simulink model "TV_2018_HIL"  (R2016a)
settings: Solver=FixedStepAuto  StartTime=0.0  StopTime=inf  FixedStep=0.001  RelTol=1e-3
PreLoadFcn:
  | TV_2017_parameters
values from neighbouring files (symbols this model uses):
  battery_voltage = single(530)    [HIL_parameters.m]    (also in HIL_parameters_2018.m; TV_2017_parameters.m; TV_2017_parameters_VD.m)
  car_params = Simulink_Car_params    [HIL_parameters.m]    (also in HIL_parameters_2018.m; TV_2017_parameters.m; TV_2017_parameters_VD.m)
  i_Diff = 16    [HIL_parameters.m]    (also in HIL_parameters_2018.m; TV_2017_parameters.m)
  Kp = 1    [HIL_parameters.m]    (also in HIL_parameters_2018.m; TV_2017_parameters.m; TV_2017_parameters_VD.m)
  motor_data = struct    [HIL_parameters.m]    (also in HIL_parameters_2018.m; TV_2017_parameters.m)
  powerLimitControl = Simulink_el    [HIL_parameters.m]    (also in HIL_parameters_2018.m; TV_2017_parameters.m; TV_2017_parameters_VD.m)
  settings = Simulink_Settings    [HIL_parameters.m]    (also in HIL_parameters_2018.m; TV_2017_parameters.m; TV_2017_parameters_VD.m)
  SpdC_BCC = 0    [HIL_parameters.m]    (also in HIL_parameters_2018.m; TV_2017_parameters.m; TV_2017_parameters_VD.m)
  Speed_Neg_sat = -21    [HIL_parameters.m]    (also in HIL_parameters_2018.m; TV_2017_parameters.m; TV_2017_parameters_VD.m)
  Speed_Pos_sat = 21    [HIL_parameters.m]    (also in HIL_parameters_2018.m; TV_2017_parameters.m; TV_2017_parameters_VD.m)
  SteeringAngleFL = [-23.80 -22.65 -21.50 -20.34 -19.18 -18.03 -16.86 -15.70 -14.53 -13.35 -12.18 -10.99 -9.80 -8.61 -7.40 -6.19 -4.97 -3.75 -2.51 -1.26 0 1.27 2.56 3.85 5.17 6.50 7.84 9.21 10.59 12.00 13.42 14.88 16.36 17.87 19.41 20.99 22.61 24.26 25.97 27.73 29.54]    [CarSetupAnalysis2018.m]    (also in HIL_parameters_2018.m; TV_2017_parameters.m; TV_2017_parameters_VD.m = [-24.129 -22.950 -21.772 -20.593 -19.413 -18.232 -17.050 -15)
  SteeringAngleFR = [-29.54 -27.73 -25.97 -24.26 -22.61 -20.99 -19.41 -17.87 -16.36 -14.88 -13.42 -12.00 -10.59 -9.21 -7.84 -6.50 -5.17 -3.85 -2.56 -1.27 0 1.26 2.51 3.75 4.97 6.19 7.40 8.61 9.80 10.99 12.18 13.35 14.53 15.70 16.86 18.03 19.18 20.34 21.50 22.65 23.80]    [CarSetupAnalysis2018.m]    (also in HIL_parameters_2018.m; TV_2017_parameters.m; TV_2017_parameters_VD.m = [-29.3050 -27.5340 -25.8140 -24.1410 -22.5110 -20.9180 -19.3)
  SteeringWhAngle = [-105 -99.75 -94.5 -89.25 -84 -78.75 -73.5 -68.25 -63 -57.75 -52.5 -47.25 -42 -36.75 -31.5 -26.25 -21.0 -15.75 -10.5 -5.25 0.0 5.25 10.50 15.75 21.00 26.25 31.50 36.75 42.00 47.25 52.50 57.75  63.00 68.25 73.50 78.75 84.00 89.25 94.50 99.75 105.00]    [TV_2017_parameters_VD.m]
  Tn_n = 0    [HIL_parameters.m]    (also in HIL_parameters_2018.m; TV_2017_parameters.m; TV_2017_parameters_VD.m)
  tractionControl = Simulink_tc    [HIL_parameters.m]    (also in HIL_parameters_2018.m; IterativeTractionControlTuning.m; TV_2017_parameters.m; TV_2017_parameters_VD.m)
  yawMomentGenerator = struct    [HIL_parameters.m]    (also in HIL_parameters_2018.m = Simulink_yawRate2; TV_2017_parameters.m = Simulink_yawRate2)
  yawRateControl = Simulink_yawRate    [HIL_parameters.m]    (also in HIL_parameters_2018.m; TV_2017_parameters.m; TV_2017_parameters_VD.m)
undefined symbols (not defined in the file or in its folder): canChannel, DiscIntNeverNeededParam, magnitude, speedEstimation, TC_Decr_Gas, TC_Derivative, TC_Incr_Gas, TC_On, TC_Relay_Off, TC_Relay_On
libraries: CarMaker4SL x366, simulink_extras x63, canmsglib x55, canlib x41, simulink x37, dspfdesign x2, sldrtlib x1
(part 7 of 15)

== system TV_2018_HIL/CarMaker/IPG Vehicle3/CarAndTrailer/Forces/Tires ==
  note: The TireXX_Out signals will only be used if FileIdent is "CarMaker-Tire-CM4SL" in the tire parameter file!
      | An example parameter file can be found in Data/Tire/DT_CM4SL_UserTire.
  Sync_In : Inport
  TireFL_In : Inport  Port=2
  TireFR_In : Inport  Port=3
  TireRL_In : Inport  Port=4
  TireRR_In : Inport  Port=5
  Bus Creator{1..4} (4 alike) : BusCreator  Inputs=11
  Demux{1..3,8} (4 alike) : Demux  Outputs=7
  Scope : Scope
  TireFL : Subsystem
  TireFR : Subsystem
  TireRL : Subsystem
  TireRR : Subsystem
  TireFL_Out : Outport
  TireFR_Out : Outport  Port=2
  TireRL_Out : Outport  Port=3
  TireRR_Out : Outport  Port=4
  wires:
  Sync_In/1 -> TireRR/1(Sync_In), TireRL/1(Sync_In), TireFR/1(Sync_In), TireFL/1(Sync_In)
  Bus Creator4/1 -> TireRR_Out/1
  Bus Creator2/1 -> TireRL_Out/1
  Bus Creator1/1 -> TireFR_Out/1
  Demux3/5 -> TireRR/6(Rim_turnv)  "Tire_In Rim_turnv"
  Demux3/4 -> TireRR/5(Rim_rotv)  "Tire_In Rim_rotv"
  Demux3/1 -> TireRR/2(Load)  "Tire_In Load"
  Demux3/7 -> TireRR/8(muRoad)  "Tire_In mu"
  Demux3/6 -> TireRR/7(InclinAngle)  "Tire_In Camber"
  Demux3/2 -> TireRR/3(vxtrans)  "Tire_In vxtrans"
  Demux3/3 -> TireRR/4(vytrans)  "Tire_In vytrans"
  TireRR/11(AlignTrq) -> Bus Creator4/11  "Tire_Out AlignTrq"
  TireRR/10(RollResist) -> Bus Creator4/10  "Tire_Out RollResist"
  TireRR/9(OverturnTrq) -> Bus Creator4/9  "Tire_Out OverturnTrq"
  TireRR/8(LoadFrc) -> Bus Creator4/8  "Tire_Out LoadFrc"
  TireRR/7(SideFrc) -> Bus Creator4/7  "Tire_Out SideFrc"
  TireRR/6(LongFrc) -> Bus Creator4/6  "Tire_Out LongFrc"
  TireRR/5(vBelt) -> Bus Creator4/5  "Tire_Out vBelt"
  TireRR/4(rBelt_eff) -> Bus Creator4/4  "Tire_Out rBelt_eff"
  TireRR/3(TurnSlp) -> Bus Creator4/3  "Tire_Out TurnSlp"
  TireRR/1(Slp) -> Bus Creator4/1  "Tire_Out Slp"
  TireRR/2(Alpha) -> Bus Creator4/2  "Tire_Out Alpha"
  Demux2/5 -> TireRL/6(Rim_turnv)  "Tire_In Rim_turnv"
  Demux2/4 -> TireRL/5(Rim_rotv)  "Tire_In Rim_rotv"
  Demux2/1 -> TireRL/2(Load)  "Tire_In Load"
  Demux2/7 -> TireRL/8(muRoad)  "Tire_In mu"
  Demux2/6 -> TireRL/7(InclinAngle)  "Tire_In Camber"
  Demux2/2 -> TireRL/3(vxtrans)  "Tire_In vxtrans"
  Demux2/3 -> TireRL/4(vytrans)  "Tire_In vytrans"
  TireRL/11(AlignTrq) -> Bus Creator2/11  "Tire_Out AlignTrq"
  TireRL/10(RollResist) -> Bus Creator2/10  "Tire_Out RollResist"
  TireRL/9(OverturnTrq) -> Bus Creator2/9  "Tire_Out OverturnTrq"
  TireRL/8(LoadFrc) -> Bus Creator2/8  "Tire_Out LoadFrc"
  TireRL/7(SideFrc) -> Bus Creator2/7  "Tire_Out SideFrc"
  TireRL/6(LongFrc) -> Bus Creator2/6  "Tire_Out LongFrc"
  TireRL/5(vBelt) -> Bus Creator2/5  "Tire_Out vBelt"
  TireRL/4(rBelt_eff) -> Bus Creator2/4  "Tire_Out rBelt_eff"
  TireRL/3(TurnSlp) -> Bus Creator2/3  "Tire_Out TurnSlp"
  TireRL/1(Slp) -> Bus Creator2/1  "Tire_Out Slp"
  TireRL/2(Alpha) -> Bus Creator2/2  "Tire_Out Alpha"
  Demux1/5 -> TireFR/6(Rim_turnv)  "Tire_In Rim_turnv"
  Demux1/4 -> TireFR/5(Rim_rotv)  "Tire_In Rim_rotv"
  Demux1/1 -> TireFR/2(Load)  "Tire_In Load"
  Demux1/7 -> TireFR/8(muRoad)  "Tire_In mu"
  Demux1/6 -> TireFR/7(InclinAngle)  "Tire_In Camber"
  Demux1/2 -> TireFR/3(vxtrans)  "Tire_In vxtrans"
  Demux1/3 -> TireFR/4(vytrans)  "Tire_In vytrans"
  TireFR/11(AlignTrq) -> Bus Creator1/11  "Tire_Out AlignTrq"
  TireFR/10(RollResist) -> Bus Creator1/10  "Tire_Out RollResist"
  TireFR/9(OverturnTrq) -> Bus Creator1/9  "Tire_Out OverturnTrq"
  TireFR/8(LoadFrc) -> Bus Creator1/8  "Tire_Out LoadFrc"
  TireFR/7(SideFrc) -> Bus Creator1/7  "Tire_Out SideFrc"
  TireFR/6(LongFrc) -> Bus Creator1/6  "Tire_Out LongFrc"
  TireFR/5(vBelt) -> Bus Creator1/5  "Tire_Out vBelt"
  TireFR/4(rBelt_eff) -> Bus Creator1/4  "Tire_Out rBelt_eff"
  TireFR/3(TurnSlp) -> Bus Creator1/3  "Tire_Out TurnSlp"
  TireFR/1(Slp) -> Bus Creator1/1  "Tire_Out Slp"
  TireFR/2(Alpha) -> Bus Creator1/2  "Tire_Out Alpha"
  Demux8/5 -> TireFL/6(Rim_turnv)  "Tire_In Rim_turnv"
  Demux8/4 -> TireFL/5(Rim_rotv)  "Tire_In Rim_rotv"
  TireFL_In/1 -> Demux8/1
  Demux8/1 -> TireFL/2(Load)  "Tire_In Load"
  Demux8/7 -> Scope/1, TireFL/8(muRoad)  "Tire_In mu"
  Demux8/6 -> TireFL/7(InclinAngle)  "Tire_In Camber"
  Demux8/2 -> TireFL/3(vxtrans)  "Tire_In vxtrans"
  Demux8/3 -> TireFL/4(vytrans)  "Tire_In vytrans"
  TireFL/11(AlignTrq) -> Bus Creator3/11  "Tire_Out AlignTrq"
  TireFL/10(RollResist) -> Bus Creator3/10  "Tire_Out RollResist"
  TireFL/9(OverturnTrq) -> Bus Creator3/9  "Tire_Out OverturnTrq"
  TireFL/8(LoadFrc) -> Bus Creator3/8  "Tire_Out LoadFrc"
  TireFL/7(SideFrc) -> Bus Creator3/7  "Tire_Out SideFrc"
  TireFL/6(LongFrc) -> Bus Creator3/6  "Tire_Out LongFrc"
  TireFL/5(vBelt) -> Bus Creator3/5  "Tire_Out vBelt"
  TireFL/4(rBelt_eff) -> Bus Creator3/4  "Tire_Out rBelt_eff"
  TireFL/3(TurnSlp) -> Bus Creator3/3  "Tire_Out TurnSlp"
  TireFL/1(Slp) -> Bus Creator3/1  "Tire_Out Slp"
  TireFL/2(Alpha) -> Bus Creator3/2  "Tire_Out Alpha"
  Bus Creator3/1 -> TireFL_Out/1
  TireFR_In/1 -> Demux1/1
  TireRL_In/1 -> Demux2/1
  TireRR_In/1 -> Demux3/1

== system TV_2018_HIL/CarMaker/IPG Vehicle3/CarAndTrailer/Forces/Vehicle Forces ==
  Sync_In : Inport
  Aero R18 prelim : Subsystem
  Bus Creator1 : BusCreator  Inputs=12
  Bus Creator8 : BusCreator  Inputs=16
  BusCreator1 : BusCreator  Inputs=4
  BusCreator2 : BusCreator  Inputs=9
  Demux : Demux  Outputs=16
  Demux1 : Demux  Outputs=12
  Demux2 : Demux  Outputs=13
  Forces : S-Function  FunctionName=CM_Sfun  Parameters='Forces'  SFunctionDeploymentMode=off  EnableBusSupport=off
  Terminator : Terminator
  Sync_Out : Outport
  Car.Virtual : Outport  Port=2
  Car.Aero : Outport  Port=3
  Car.Load : Outport  Port=4
  wires:
  BusCreator1/1 -> Terminator/1  "Aero IF (in)"
  Demux/16 -> Bus Creator8/16  "Car Load_3 tz"
  Demux/15 -> Bus Creator8/15  "Car Load_3 ty"
  Demux/14 -> Bus Creator8/14  "Car Load_3 tx"
  Demux/13 -> Bus Creator8/13  "Car Load_3 mass"
  Demux1/12 -> Bus Creator1/12  "Car Virtual Trq_0 z"
  Demux1/11 -> Bus Creator1/11  "Car Virtual Trq_0 y"
  Demux1/10 -> Bus Creator1/10  "Car Virtual Trq_0 x"
  Demux1/9 -> Bus Creator1/9  "Car Virtual Trq_1 z"
  Demux1/8 -> Bus Creator1/8  "Car Virtual Trq_1 y"
  Demux1/7 -> Bus Creator1/7  "Car Virtual Trq_1 x"
  Demux1/6 -> Bus Creator1/6  "Car Virtual Frc_0 z"
  Demux1/5 -> Bus Creator1/5  "Car Virtual Frc_0 y"
  Demux1/4 -> Bus Creator1/4  "Car Virtual Frc_0 x"
  Sync_In/1 -> Forces/1
  Forces/1 -> Sync_Out/1
  BusCreator2/1 -> Car.Aero/1
  Demux1/1 -> Bus Creator1/1  "Car Virtual Frc_1 x"
  Demux1/2 -> Bus Creator1/2  "Car Virtual Frc_1 y"
  Demux1/3 -> Bus Creator1/3  "Car Virtual Frc_1 z"
  Forces/3 -> Demux2/1
  Forces/2 -> Demux1/1
  Bus Creator1/1 -> Car.Virtual/1
  Bus Creator8/1 -> Car.Load/1
  Demux/1 -> Bus Creator8/1  "Car Load_0 mass"
  Demux/2 -> Bus Creator8/2  "Car Load_0 tx"
  Demux/3 -> Bus Creator8/3  "Car Load_0 ty"
  Demux/4 -> Bus Creator8/4  "Car Load_0 tz"
  Demux/5 -> Bus Creator8/5  "Car Load_1 mass"
  Demux/6 -> Bus Creator8/6  "Car Load_1 tx"
  Demux/7 -> Bus Creator8/7  "Car Load_1 ty"
  Demux/8 -> Bus Creator8/8  "Car Load_1 tz"
  Demux/9 -> Bus Creator8/9  "Car Load_2 mass"
  Demux/10 -> Bus Creator8/10  "Car Load_2 tx"
  Demux/11 -> Bus Creator8/11  "Car Load_2 ty"
  Demux/12 -> Bus Creator8/12  "Car Load_2 tz"
  Forces/4 -> Demux/1
  Demux2/1 -> Aero R18 prelim/1(car Aero ApproachVel_1 x)  "car Aero ApproachVel_1 x"
  Demux2/2 -> Aero R18 prelim/2(car Aero ApproachVel_1 y)  "car Aero ApproachVel_1 y"
  Demux2/3 -> Aero R18 prelim/3(car Aero ApproachVel_1 z)  "car Aero ApproachVel_1 z"
  Demux2/4 -> Aero R18 prelim/4(car Aero tau_1)  "car Aero tau_1"
  Demux2/5 -> Aero R18 prelim/5(car Aero PoA_1 x)  "car Aero PoA_1 x"
  Demux2/6 -> Aero R18 prelim/6(car Aero PoA_1 y)  "car Aero PoA_1 y"
  Demux2/7 -> Aero R18 prelim/7(car Aero PoA_1 z)  "car Aero PoA_1 z"
  Demux2/8 -> Aero R18 prelim/8(car Aero Frc_1 x)  "car Aero Frc_1 x"
  Demux2/9 -> Aero R18 prelim/9(car Aero Frc_1 y)  "car Aero Frc_1 y"
  Demux2/10 -> Aero R18 prelim/10(car Aero Frc_1 z)  "car Aero Frc_1 z"
  Demux2/11 -> Aero R18 prelim/11(car Aero Trq_1 x)  "car Aero Trq_1 x"
  Demux2/12 -> Aero R18 prelim/12(car Aero Trq_1 y)  "car Aero Trq_1 y"
  Demux2/13 -> Aero R18 prelim/13(car Aero Trq_1 z)  "car Aero Trq_1 z"
  Aero R18 prelim/7(car Aero PoA_1 z_R18) -> BusCreator2/3
  Aero R18 prelim/8(car Aero Frc_1 x_R18) -> BusCreator2/4
  Aero R18 prelim/9(car Aero Frc_1 y_R18) -> BusCreator2/5
  Aero R18 prelim/10(car Aero Frc_1 z_R18) -> BusCreator2/6
  Aero R18 prelim/11(car Aero Trq_1 x_R18) -> BusCreator2/7
  Aero R18 prelim/12(car Aero Trq_1 y_R18) -> BusCreator2/8
  Aero R18 prelim/13(car Aero Trq_1 z_R18) -> BusCreator2/9
  Aero R18 prelim/5(car Aero PoA_1 x_R18) -> BusCreator2/1
  Aero R18 prelim/6(car Aero PoA_1 y_R18) -> BusCreator2/2
  Aero R18 prelim/4(car Aero tau_1_R18) -> BusCreator1/4
  Aero R18 prelim/3(car Aero ApproachVel_1 z_R18) -> BusCreator1/3
  Aero R18 prelim/2(car Aero ApproachVel_1 y_R18) -> BusCreator1/2
  Aero R18 prelim/1(car Aero ApproachVel_1 x_R18) -> BusCreator1/1

== system TV_2018_HIL/CarMaker/IPG Vehicle3/CarAndTrailer/Trailer/CreateBus Car.Hitch.FrcTrq ==
  In1 : Inport
  Bus Creator7 : BusCreator  Inputs=6
  Demux7 : Demux  Outputs=6
  Out1 : Outport
  wires:
  In1/1 -> Demux7/1
  Bus Creator7/1 -> Out1/1
  Demux7/6 -> Bus Creator7/6  "Car Hitch Trq2Car z"
  Demux7/5 -> Bus Creator7/5  "Car Hitch Trq2Car y"
  Demux7/4 -> Bus Creator7/4  "Car Hitch Trq2Car x"
  Demux7/3 -> Bus Creator7/3  "Car Hitch Frc2Car z"
  Demux7/2 -> Bus Creator7/2  "Car Hitch Frc2Car y"
  Demux7/1 -> Bus Creator7/1  "Car Hitch Frc2Car x"

== system TV_2018_HIL/CarMaker/IPG Vehicle3/CarAndTrailer/Trailer/CreateBus Vhcl.Motion ==
  In1 : Inport
  BusCreator : BusCreator  Inputs=15
  Demux : Demux  Outputs=15
  Out1 : Outport
  wires:
  Demux/15 -> BusCreator/15  "Vhcl YawAcc"
  Demux/14 -> BusCreator/14  "Vhcl YawVel"
  Demux/13 -> BusCreator/13  "Vhcl Yaw"
  Demux/12 -> BusCreator/12  "Vhcl PitchAcc"
  Demux/11 -> BusCreator/11  "Vhcl PitchVel"
  Demux/10 -> BusCreator/10  "Vhcl Pitch"
  Demux/9 -> BusCreator/9  "Vhcl RollAcc"
  Demux/8 -> BusCreator/8  "Vhcl RollVel"
  Demux/7 -> BusCreator/7  "Vhcl Roll"
  Demux/6 -> BusCreator/6  "Vhcl Hitch_Pos z"
  Demux/5 -> BusCreator/5  "Vhcl Hitch_Pos y"
  Demux/4 -> BusCreator/4  "Vhcl Hitch_Pos x"
  Demux/3 -> BusCreator/3  "Vhcl sRoad"
  Demux/2 -> BusCreator/2  "Vhcl Distance"
  Demux/1 -> BusCreator/1  "Vhcl v"
  In1/1 -> Demux/1
  BusCreator/1 -> Out1/1

== system TV_2018_HIL/CarMaker/IPG Vehicle3/CarAndTrailer/Trailer/CreateBus Vhcl.PoI ==
  In1 : Inport
  Bus Creator3 : BusCreator  Inputs=18
  Demux3 : Demux  Outputs=18
  Out1 : Outport
  wires:
  Demux3/18 -> Bus Creator3/18  "Vhcl PoI_GCS Elev"
  Demux3/17 -> Bus Creator3/17  "Vhcl PoI_GCS Lat"
  Demux3/16 -> Bus Creator3/16  "Vhcl PoI_GCS Long"
  Demux3/15 -> Bus Creator3/15  "Vhcl PoI_Acc_1 z"
  Demux3/14 -> Bus Creator3/14  "Vhcl PoI_Acc_1 y"
  Demux3/13 -> Bus Creator3/13  "Vhcl PoI_Acc_1 x"
  Demux3/12 -> Bus Creator3/12  "Vhcl PoI_Vel_1 z"
  Demux3/11 -> Bus Creator3/11  "Vhcl PoI_Vel_1 y"
  Demux3/10 -> Bus Creator3/10  "Vhcl PoI_Vel_1 x"
  Demux3/9 -> Bus Creator3/9  "Vhcl PoI_Acc z"
  Demux3/8 -> Bus Creator3/8  "Vhcl PoI_Acc y"
  Demux3/7 -> Bus Creator3/7  "Vhcl PoI_Acc x"
  Demux3/6 -> Bus Creator3/6  "Vhcl PoI_Vel z"
  Demux3/5 -> Bus Creator3/5  "Vhcl PoI_Vel y"
  Demux3/4 -> Bus Creator3/4  "Vhcl PoI_Vel x"
  Demux3/3 -> Bus Creator3/3  "Vhcl PoI_Pos z"
  Demux3/2 -> Bus Creator3/2  "Vhcl PoI_Pos y"
  In1/1 -> Demux3/1
  Bus Creator3/1 -> Out1/1
  Demux3/1 -> Bus Creator3/1  "Vhcl PoI_Pos x"

== system TV_2018_HIL/CarMaker/IPG Vehicle3/CarAndTrailer/Trailer/CreateBus Vhcl.Steering ==
  In1 : Inport
  Bus Creator3 : BusCreator  Inputs=4
  Demux : Demux
  Out1 : Outport
  wires:
  Bus Creator3/1 -> Out1/1
  Demux/1 -> Bus Creator3/1  "Vhcl Steering Ang"
  Demux/3 -> Bus Creator3/3  "Vhcl Steering AngAcc"
  Demux/2 -> Bus Creator3/2  "Vhcl Steering AngVel"
  Demux/4 -> Bus Creator3/4  "Vhcl Steering Trq"
  In1/1 -> Demux/1

== system TV_2018_HIL/CarMaker/IPG Vehicle3/CarAndTrailer/Trailer/CreateBus Vhcl.Wheel.FL ==
  In1 : Inport
  Bus Creator3 : BusCreator  Inputs=14
  Demux3 : Demux  Outputs=14
  Out1 : Outport
  wires:
  Demux3/14 -> Bus Creator3/14  "Vhcl Wheel FL Trq_WhlBearing"
  Demux3/13 -> Bus Creator3/13  "Vhcl Wheel FL Trq_T2W"
  Demux3/12 -> Bus Creator3/12  "Vhcl Wheel FL SideSlip"
  Demux3/11 -> Bus Creator3/11  "Vhcl Wheel FL LongSlip"
  Demux3/10 -> Bus Creator3/10  "Vhcl Wheel FL vBelt"
  Demux3/9 -> Bus Creator3/9  "Vhcl Wheel FL Fz"
  Demux3/8 -> Bus Creator3/8  "Vhcl Wheel FL Fy"
  Demux3/7 -> Bus Creator3/7  "Vhcl Wheel FL Fx"
  Demux3/6 -> Bus Creator3/6  "Vhcl Wheel FL r_zxy z"
  Demux3/5 -> Bus Creator3/5  "Vhcl Wheel FL r_zxy y"
  Demux3/4 -> Bus Creator3/4  "Vhcl Wheel FL r_zxy x"
  Demux3/3 -> Bus Creator3/3  "Vhcl Wheel FL t z"
  Demux3/2 -> Bus Creator3/2  "Vhcl Wheel FL t y"
  In1/1 -> Demux3/1
  Bus Creator3/1 -> Out1/1
  Demux3/1 -> Bus Creator3/1  "Vhcl Wheel FL t x"

== system TV_2018_HIL/CarMaker/IPG Vehicle3/CarAndTrailer/Trailer/CreateBus Vhcl.Wheel.FR ==
  In1 : Inport
  Bus Creator3 : BusCreator  Inputs=14
  Demux3 : Demux  Outputs=14
  Out1 : Outport
  wires:
  Demux3/14 -> Bus Creator3/14  "Vhcl Wheel FR Trq_WhlBearing"
  Demux3/13 -> Bus Creator3/13  "Vhcl Wheel FR Trq_T2W"
  Demux3/12 -> Bus Creator3/12  "Vhcl Wheel FR SideSlip"
  Demux3/11 -> Bus Creator3/11  "Vhcl Wheel FR LongSlip"
  Demux3/10 -> Bus Creator3/10  "Vhcl Wheel FR vBelt"
  Demux3/9 -> Bus Creator3/9  "Vhcl Wheel FR Fz"
  Demux3/8 -> Bus Creator3/8  "Vhcl Wheel FR Fy"
  Demux3/7 -> Bus Creator3/7  "Vhcl Wheel FR Fx"
  Demux3/6 -> Bus Creator3/6  "Vhcl Wheel FR r_zxy z"
  Demux3/5 -> Bus Creator3/5  "Vhcl Wheel FR r_zxy y"
  Demux3/4 -> Bus Creator3/4  "Vhcl Wheel FR r_zxy x"
  Demux3/3 -> Bus Creator3/3  "Vhcl Wheel FR t z"
  Demux3/2 -> Bus Creator3/2  "Vhcl Wheel FR t y"
  In1/1 -> Demux3/1
  Bus Creator3/1 -> Out1/1
  Demux3/1 -> Bus Creator3/1  "Vhcl Wheel FR t x"

== system TV_2018_HIL/CarMaker/IPG Vehicle3/CarAndTrailer/Trailer/CreateBus Vhcl.Wheel.RL ==
  In1 : Inport
  Bus Creator3 : BusCreator  Inputs=14
  Demux3 : Demux  Outputs=14
  Out1 : Outport
  wires:
  Demux3/14 -> Bus Creator3/14  "Vhcl Wheel RL Trq_WhlBearing"
  Demux3/13 -> Bus Creator3/13  "Vhcl Wheel RL Trq_T2W"
  Demux3/12 -> Bus Creator3/12  "Vhcl Wheel RL SideSlip"
  Demux3/11 -> Bus Creator3/11  "Vhcl Wheel RL LongSlip"
  Demux3/10 -> Bus Creator3/10  "Vhcl Wheel RL vBelt"
  Demux3/9 -> Bus Creator3/9  "Vhcl Wheel RL Fz"
  Demux3/8 -> Bus Creator3/8  "Vhcl Wheel RL Fy"
  Demux3/7 -> Bus Creator3/7  "Vhcl Wheel RL Fx"
  Demux3/6 -> Bus Creator3/6  "Vhcl Wheel RL r_zxy z"
  Demux3/5 -> Bus Creator3/5  "Vhcl Wheel RL r_zxy y"
  Demux3/4 -> Bus Creator3/4  "Vhcl Wheel RL r_zxy x"
  Demux3/3 -> Bus Creator3/3  "Vhcl Wheel RL t z"
  Demux3/2 -> Bus Creator3/2  "Vhcl Wheel RL t y"
  In1/1 -> Demux3/1
  Bus Creator3/1 -> Out1/1
  Demux3/1 -> Bus Creator3/1  "Vhcl Wheel RL t x"

== system TV_2018_HIL/CarMaker/IPG Vehicle3/CarAndTrailer/Trailer/CreateBus Vhcl.Wheel.RR ==
  In1 : Inport
  Bus Creator3 : BusCreator  Inputs=14
  Demux3 : Demux  Outputs=14
  Out1 : Outport
  wires:
  Demux3/14 -> Bus Creator3/14  "Vhcl Wheel RR Trq_WhlBearing"
  Demux3/13 -> Bus Creator3/13  "Vhcl Wheel RR Trq_T2W"
  Demux3/12 -> Bus Creator3/12  "Vhcl Wheel RR SideSlip"
  Demux3/11 -> Bus Creator3/11  "Vhcl Wheel RR LongSlip"
  Demux3/10 -> Bus Creator3/10  "Vhcl Wheel RR vBelt"
  Demux3/9 -> Bus Creator3/9  "Vhcl Wheel RR Fz"
  Demux3/8 -> Bus Creator3/8  "Vhcl Wheel RR Fy"
  Demux3/7 -> Bus Creator3/7  "Vhcl Wheel RR Fx"
  Demux3/6 -> Bus Creator3/6  "Vhcl Wheel RR r_zxy z"
  Demux3/5 -> Bus Creator3/5  "Vhcl Wheel RR r_zxy y"
  Demux3/4 -> Bus Creator3/4  "Vhcl Wheel RR r_zxy x"
  Demux3/3 -> Bus Creator3/3  "Vhcl Wheel RR t z"
  Demux3/2 -> Bus Creator3/2  "Vhcl Wheel RR t y"
  In1/1 -> Demux3/1
  Bus Creator3/1 -> Out1/1
  Demux3/1 -> Bus Creator3/1  "Vhcl Wheel RR t x"

== system TV_2018_HIL/CarMaker/IPG Vehicle3/PowerTrain/Electric Powertrain/AMK FL ==
  Motor_speed_ref_in_RPM : Inport
  Whl_speed_rad_per_sec : Inport  Port=2
  "Torque_limit_pos " : Inport  Port=3
  Torque_limit_neg : Inport  Port=4
  Convert to RPM : Gain  Gain=60/(2*pi)
  Delay : Delay  DelayLength=3  InitialCondition=0
  Gain2 : Gain  Gain=-1
  Gear ratio : Gain  Gain=car_params.GR
  Gear ratio2 : Gain  Gain=car_params.GR
  Maximum torque output based on motor RPM : Lookup_n-D  NumberOfTableDimensions=1  BreakpointsForDimension1=motor_data.MaxTorqueBreakpoints  BreakpointsForDimension1Min=[0]  BreakpointsForDimension1Max=[20000]  Table=motor_data.MaxTorqueValues  ExtrapMethod=Clip  UseLastTableValue=on  InternalRulePriority=Speed  OutMin=[0]  OutMax=[21]  RndMeth=Simplest  InputSameDT=on
  Saturation : simulink/Discontinuities/Saturation Dynamic  OutMin=[]  OutMax=[]  OutDataTypeStr=Inherit: Same as second input  OutDataType=fixdt(1, 16)  OutScaling=2^-10  DoSatur=off
  Saturation Dynamic1 : simulink/Discontinuities/Saturation Dynamic  OutMin=[]  OutMax=[]  OutDataTypeStr=Inherit: Same as second input  OutDataType=fixdt(1, 16)  OutScaling=2^-10  DoSatur=off
  Speed PI 1 : simulink/Continuous/PID Controller  Controller=PI  TimeDomain=Discrete-time  SampleTime=-1  IntegratorMethod=Forward Euler  FilterMethod=Forward Euler  Form=Parallel  UseFilter=on  ControllerParametersSource=internal  P=Kp  I=Tn_n  D=0  N=100  InitialConditionSource=internal  InitialConditionForIntegrator=0  InitialConditionForFilter=0  ExternalReset=none  LimitOutput=on  UpperSaturationLimit=Speed_Pos_sat  LowerSaturationLimit=Speed_Neg_sat  LinearizeAsGain=off  AntiWindupMode=back-calculation  Kb=SpdC_BCC  TrackingMode=off  Kt=1  PParamMin=[]  PParamMax=[]  IParamMin=[]  IParamMax=[]  DParamMin=[]  DParamMax=[]  NParamMin=[]  NParamMax=[]  KbParamMin=[]  KbParamMax=[]  KtParamMin=[]  KtParamMax=[]  POutMin=[]  POutMax=[]  IOutMin=[]  IOutMax=[]  DOutMin=[]  DOutMax=[]  NOutMin=[]  NOutMax=[]  KbOutMin=[]  KbOutMax=[]  KtOutMin=[]  KtOutMax=[]  IntegratorOutMin=[]  IntegratorOutMax=[]  FilterOutMin=[]  FilterOutMax=[]  SumOutMin=[]  SumOutMax=[]  SumI1OutMin=[]  SumI1OutMax=[]  SumI2OutMin=[]  SumI2OutMax=[]  SumI3OutMin=[]  SumI3OutMax=[]  SumDOutMin=[]  SumDOutMax=[]  SaturationOutMin=[]  SaturationOutMax=[]  IntegratorContinuousStateAttributes=''  IntegratorStateMustResolveToSignalObject=off  IntegratorRTWStateStorageClass=Auto  FilterContinuousStateAttributes=''  FilterStateMustResolveToSignalObject=off  FilterRTWStateStorageClass=Auto  DifferentiatorICPrevScaledInput=0  DifferentiatorOutMin=[]  DifferentiatorOutMax=[]
  Sum : Sum  Inputs=|+-
  "Torque_output_at_wheel " : Outport
  wires:
  Gear ratio/1 -> Convert to RPM/1
  Convert to RPM/1 -> Maximum torque output based on motor RPM/1, Sum/2
  Sum/1 -> Speed PI 1/1
  Saturation/1 -> Saturation Dynamic1/2
  Motor_speed_ref_in_RPM/1 -> Sum/1
  Torque_limit_neg/1 -> Saturation/3
  "Torque_limit_pos "/1 -> Saturation/1
  Gear ratio2/1 -> Delay/1
  Gain2/1 -> Saturation Dynamic1/3
  Whl_speed_rad_per_sec/1 -> Gear ratio/1
  Saturation Dynamic1/1 -> Gear ratio2/1
  Maximum torque output based on motor RPM/1 -> Gain2/1, Saturation Dynamic1/1
  Speed PI 1/1 -> Saturation/2
  Delay/1 -> "Torque_output_at_wheel "/1

== system TV_2018_HIL/CarMaker/IPG Vehicle3/PowerTrain/Electric Powertrain/AMK FR ==
  Motor_speed_ref_in_RPM : Inport
  Whl_speed_rad_per_sec : Inport  Port=2
  "Torque_limit_pos " : Inport  Port=3
  Torque_limit_neg : Inport  Port=4
  Convert to RPM : Gain  Gain=60/(2*pi)
  Delay : Delay  DelayLength=3  InitialCondition=0
  Gain2 : Gain  Gain=-1
  Gear ratio : Gain  Gain=car_params.GR
  Gear ratio2 : Gain  Gain=car_params.GR
  Maximum torque output based on motor RPM : Lookup_n-D  NumberOfTableDimensions=1  BreakpointsForDimension1=motor_data.MaxTorqueBreakpoints  BreakpointsForDimension1Min=[0]  BreakpointsForDimension1Max=[20000]  Table=motor_data.MaxTorqueValues  ExtrapMethod=Clip  UseLastTableValue=on  InternalRulePriority=Speed  OutMin=[0]  OutMax=[21]  RndMeth=Simplest  InputSameDT=on
  Saturation : simulink/Discontinuities/Saturation Dynamic  OutMin=[]  OutMax=[]  OutDataTypeStr=Inherit: Same as second input  OutDataType=fixdt(1, 16)  OutScaling=2^-10  DoSatur=off
  Saturation Dynamic1 : simulink/Discontinuities/Saturation Dynamic  OutMin=[]  OutMax=[]  OutDataTypeStr=Inherit: Same as second input  OutDataType=fixdt(1, 16)  OutScaling=2^-10  DoSatur=off
  Speed PI 1 : simulink/Continuous/PID Controller  Controller=PI  TimeDomain=Discrete-time  SampleTime=-1  IntegratorMethod=Forward Euler  FilterMethod=Forward Euler  Form=Parallel  UseFilter=on  ControllerParametersSource=internal  P=Kp  I=Tn_n  D=0  N=100  InitialConditionSource=internal  InitialConditionForIntegrator=0  InitialConditionForFilter=0  ExternalReset=none  ZeroCross=off  LimitOutput=on  UpperSaturationLimit=Speed_Pos_sat  LowerSaturationLimit=Speed_Neg_sat  LinearizeAsGain=off  AntiWindupMode=back-calculation  Kb=SpdC_BCC  TrackingMode=off  Kt=1  PParamMin=[]  PParamMax=[]  IParamMin=[]  IParamMax=[]  DParamMin=[]  DParamMax=[]  NParamMin=[]  NParamMax=[]  KbParamMin=[]  KbParamMax=[]  KtParamMin=[]  KtParamMax=[]  POutMin=[]  POutMax=[]  IOutMin=[]  IOutMax=[]  DOutMin=[]  DOutMax=[]  NOutMin=[]  NOutMax=[]  KbOutMin=[]  KbOutMax=[]  KtOutMin=[]  KtOutMax=[]  IntegratorOutMin=[]  IntegratorOutMax=[]  FilterOutMin=[]  FilterOutMax=[]  SumOutMin=[]  SumOutMax=[]  SumI1OutMin=[]  SumI1OutMax=[]  SumI2OutMin=[]  SumI2OutMax=[]  SumI3OutMin=[]  SumI3OutMax=[]  SumDOutMin=[]  SumDOutMax=[]  SaturationOutMin=[]  SaturationOutMax=[]  IntegratorContinuousStateAttributes=''  IntegratorStateMustResolveToSignalObject=off  IntegratorRTWStateStorageClass=Auto  FilterContinuousStateAttributes=''  FilterStateMustResolveToSignalObject=off  FilterRTWStateStorageClass=Auto  DifferentiatorICPrevScaledInput=0  DifferentiatorOutMin=[]  DifferentiatorOutMax=[]
  Sum : Sum  Inputs=|+-
  "Torque_Output " : Outport
  wires:
  Gear ratio/1 -> Convert to RPM/1
  Convert to RPM/1 -> Maximum torque output based on motor RPM/1, Sum/2
  Sum/1 -> Speed PI 1/1
  Saturation/1 -> Saturation Dynamic1/2
  Motor_speed_ref_in_RPM/1 -> Sum/1
  Torque_limit_neg/1 -> Saturation/3
  "Torque_limit_pos "/1 -> Saturation/1
  Gear ratio2/1 -> Delay/1
  Gain2/1 -> Saturation Dynamic1/3
  Whl_speed_rad_per_sec/1 -> Gear ratio/1
  Saturation Dynamic1/1 -> Gear ratio2/1
  Maximum torque output based on motor RPM/1 -> Gain2/1, Saturation Dynamic1/1
  Speed PI 1/1 -> Saturation/2
  Delay/1 -> "Torque_Output "/1

== system TV_2018_HIL/CarMaker/IPG Vehicle3/PowerTrain/Electric Powertrain/AMK RL ==
  Motor_speed_ref_in_RPM : Inport
  Whl_speed_rad_per_sec : Inport  Port=2
  "Torque_limit_pos " : Inport  Port=3
  Torque_limit_neg : Inport  Port=4
  Convert to RPM : Gain  Gain=60/(2*pi)
  Delay : Delay  DelayLength=3  InitialCondition=0
  Gain2 : Gain  Gain=-1
  Gear ratio : Gain  Gain=car_params.GR
  Gear ratio2 : Gain  Gain=car_params.GR
  Maximum torque output based on motor RPM : Lookup_n-D  NumberOfTableDimensions=1  BreakpointsForDimension1=motor_data.MaxTorqueBreakpoints  BreakpointsForDimension1Min=[0]  BreakpointsForDimension1Max=[20000]  Table=motor_data.MaxTorqueValues  ExtrapMethod=Clip  UseLastTableValue=on  InternalRulePriority=Speed  OutMin=[0]  OutMax=[21]  RndMeth=Simplest  InputSameDT=on
  Saturation : simulink/Discontinuities/Saturation Dynamic  OutMin=[]  OutMax=[]  OutDataTypeStr=Inherit: Same as second input  OutDataType=fixdt(1, 16)  OutScaling=2^-10  DoSatur=off
  Saturation Dynamic1 : simulink/Discontinuities/Saturation Dynamic  OutMin=[]  OutMax=[]  OutDataTypeStr=Inherit: Same as second input  OutDataType=fixdt(1, 16)  OutScaling=2^-10  DoSatur=off
  Speed PI 1 : simulink/Continuous/PID Controller  Controller=PI  TimeDomain=Discrete-time  SampleTime=-1  IntegratorMethod=Forward Euler  FilterMethod=Forward Euler  Form=Parallel  UseFilter=on  ControllerParametersSource=internal  P=Kp  I=Tn_n  D=0  N=100  InitialConditionSource=internal  InitialConditionForIntegrator=0  InitialConditionForFilter=0  ExternalReset=none  LimitOutput=on  UpperSaturationLimit=Speed_Pos_sat  LowerSaturationLimit=Speed_Neg_sat  LinearizeAsGain=off  AntiWindupMode=back-calculation  Kb=SpdC_BCC  TrackingMode=off  Kt=1  PParamMin=[]  PParamMax=[]  IParamMin=[]  IParamMax=[]  DParamMin=[]  DParamMax=[]  NParamMin=[]  NParamMax=[]  KbParamMin=[]  KbParamMax=[]  KtParamMin=[]  KtParamMax=[]  POutMin=[]  POutMax=[]  IOutMin=[]  IOutMax=[]  DOutMin=[]  DOutMax=[]  NOutMin=[]  NOutMax=[]  KbOutMin=[]  KbOutMax=[]  KtOutMin=[]  KtOutMax=[]  IntegratorOutMin=[]  IntegratorOutMax=[]  FilterOutMin=[]  FilterOutMax=[]  SumOutMin=[]  SumOutMax=[]  SumI1OutMin=[]  SumI1OutMax=[]  SumI2OutMin=[]  SumI2OutMax=[]  SumI3OutMin=[]  SumI3OutMax=[]  SumDOutMin=[]  SumDOutMax=[]  SaturationOutMin=[]  SaturationOutMax=[]  IntegratorContinuousStateAttributes=''  IntegratorStateMustResolveToSignalObject=off  IntegratorRTWStateStorageClass=Auto  FilterContinuousStateAttributes=''  FilterStateMustResolveToSignalObject=off  FilterRTWStateStorageClass=Auto  DifferentiatorICPrevScaledInput=0  DifferentiatorOutMin=[]  DifferentiatorOutMax=[]
  Sum : Sum  Inputs=|+-
  "Torque_Output " : Outport
  wires:
  Delay/1 -> "Torque_Output "/1
  Speed PI 1/1 -> Saturation/2
  Maximum torque output based on motor RPM/1 -> Saturation Dynamic1/1, Gain2/1
  Saturation Dynamic1/1 -> Gear ratio2/1
  Whl_speed_rad_per_sec/1 -> Gear ratio/1
  Gain2/1 -> Saturation Dynamic1/3
  Gear ratio2/1 -> Delay/1
  "Torque_limit_pos "/1 -> Saturation/1
  Torque_limit_neg/1 -> Saturation/3
  Motor_speed_ref_in_RPM/1 -> Sum/1
  Saturation/1 -> Saturation Dynamic1/2
  Sum/1 -> Speed PI 1/1
  Convert to RPM/1 -> Sum/2, Maximum torque output based on motor RPM/1
  Gear ratio/1 -> Convert to RPM/1

== system TV_2018_HIL/CarMaker/IPG Vehicle3/PowerTrain/Electric Powertrain/AMK RR ==
  Motor_speed_ref_in_RPM : Inport
  Whl_speed_rad_per_sec : Inport  Port=2
  "Torque_limit_pos " : Inport  Port=3
  Torque_limit_neg : Inport  Port=4
  Convert to RPM : Gain  Gain=60/(2*pi)
  Delay : Delay  DelayLength=3  InitialCondition=0
  Gain2 : Gain  Gain=-1
  Gear ratio : Gain  Gain=car_params.GR
  Gear ratio2 : Gain  Gain=car_params.GR
  Maximum torque output based on motor RPM : Lookup_n-D  NumberOfTableDimensions=1  BreakpointsForDimension1=motor_data.MaxTorqueBreakpoints  BreakpointsForDimension1Min=[0]  BreakpointsForDimension1Max=[20000]  Table=motor_data.MaxTorqueValues  ExtrapMethod=Clip  UseLastTableValue=on  InternalRulePriority=Speed  OutMin=[0]  OutMax=[21]  RndMeth=Simplest  InputSameDT=on
  Saturation : simulink/Discontinuities/Saturation Dynamic  OutMin=[]  OutMax=[]  OutDataTypeStr=Inherit: Same as second input  OutDataType=fixdt(1, 16)  OutScaling=2^-10  DoSatur=off
  Saturation Dynamic1 : simulink/Discontinuities/Saturation Dynamic  OutMin=[]  OutMax=[]  OutDataTypeStr=Inherit: Same as second input  OutDataType=fixdt(1, 16)  OutScaling=2^-10  DoSatur=off
  Speed PI 1 : simulink/Continuous/PID Controller  Controller=PI  TimeDomain=Discrete-time  SampleTime=-1  IntegratorMethod=Forward Euler  FilterMethod=Forward Euler  Form=Parallel  UseFilter=on  ControllerParametersSource=internal  P=Kp  I=Tn_n  D=0  N=100  InitialConditionSource=internal  InitialConditionForIntegrator=0  InitialConditionForFilter=0  ExternalReset=none  LimitOutput=on  UpperSaturationLimit=Speed_Pos_sat  LowerSaturationLimit=Speed_Neg_sat  LinearizeAsGain=off  AntiWindupMode=back-calculation  Kb=SpdC_BCC  TrackingMode=off  Kt=1  PParamMin=[]  PParamMax=[]  IParamMin=[]  IParamMax=[]  DParamMin=[]  DParamMax=[]  NParamMin=[]  NParamMax=[]  KbParamMin=[]  KbParamMax=[]  KtParamMin=[]  KtParamMax=[]  POutMin=[]  POutMax=[]  IOutMin=[]  IOutMax=[]  DOutMin=[]  DOutMax=[]  NOutMin=[]  NOutMax=[]  KbOutMin=[]  KbOutMax=[]  KtOutMin=[]  KtOutMax=[]  IntegratorOutMin=[]  IntegratorOutMax=[]  FilterOutMin=[]  FilterOutMax=[]  SumOutMin=[]  SumOutMax=[]  SumI1OutMin=[]  SumI1OutMax=[]  SumI2OutMin=[]  SumI2OutMax=[]  SumI3OutMin=[]  SumI3OutMax=[]  SumDOutMin=[]  SumDOutMax=[]  SaturationOutMin=[]  SaturationOutMax=[]  IntegratorContinuousStateAttributes=''  IntegratorStateMustResolveToSignalObject=off  IntegratorRTWStateStorageClass=Auto  FilterContinuousStateAttributes=''  FilterStateMustResolveToSignalObject=off  FilterRTWStateStorageClass=Auto  DifferentiatorICPrevScaledInput=0  DifferentiatorOutMin=[]  DifferentiatorOutMax=[]
  Sum : Sum  Inputs=|+-
  "Torque_Output " : Outport
  wires:
  Gear ratio/1 -> Convert to RPM/1
  Convert to RPM/1 -> Maximum torque output based on motor RPM/1, Sum/2
  Sum/1 -> Speed PI 1/1
  Saturation/1 -> Saturation Dynamic1/2
  Motor_speed_ref_in_RPM/1 -> Sum/1
  Torque_limit_neg/1 -> Saturation/3
  "Torque_limit_pos "/1 -> Saturation/1
  Gear ratio2/1 -> Delay/1
  Gain2/1 -> Saturation Dynamic1/3
  Whl_speed_rad_per_sec/1 -> Gear ratio/1
  Saturation Dynamic1/1 -> Gear ratio2/1
  Maximum torque output based on motor RPM/1 -> Gain2/1, Saturation Dynamic1/1
  Speed PI 1/1 -> Saturation/2
  Delay/1 -> "Torque_Output "/1

== system TV_2018_HIL/CarMaker/IPG Vehicle3/PowerTrain/Electric Powertrain/E-Gas // E-Motor ==
  VC.Gas : Inport
  Constant : Constant  Value=TC_On
  Constant1 : Constant  Value=TC_On
  E-Motor Mapping RL : Lookup2D  RowIndex=FSE_M85(1,2:end)  ColumnIndex=FSE_M85(2:end,1)  Table=FSE_M85(2:end,2:end)'  LookUpMeth=Interpolation-Use End Values
  E-Motor Mapping RR : Lookup2D  RowIndex=FSE_M85(1,2:end)  ColumnIndex=FSE_M85(2:end,1)  Table=FSE_M85(2:end,2:end)'  LookUpMeth=Interpolation-Use End Values
  Electronic Gas Pedal RL : Subsystem
  Electronic Gas Pedal RR : Subsystem
  Gain : Gain
  Gain1 : Gain
  Rotation RL : Subsystem
  Rotation RR : Subsystem
  Transfer Fcn : TransferFcn  Denominator=[0.015 1]
  Transfer Fcn1 : TransferFcn  Denominator=[0.015 1]
  Trq_RL : Outport
  Trq_RR : Outport  Port=2
  wires:
  Rotation RL/1(Engine_rot_RL) -> E-Motor Mapping RL/1
  Constant/1 -> Electronic Gas Pedal RL/1(TC_On)
  Electronic Gas Pedal RL/1(Motor_Gas_RL) -> E-Motor Mapping RL/2
  VC.Gas/1 -> Electronic Gas Pedal RL/2(VC.Gas), Electronic Gas Pedal RR/2(VC.Gas)
  Constant1/1 -> Electronic Gas Pedal RR/1(TC_On)
  E-Motor Mapping RL/1 -> Transfer Fcn/1
  Transfer Fcn/1 -> Gain/1
  Gain/1 -> Trq_RL/1
  Rotation RR/1(Engine_rot_RR) -> E-Motor Mapping RR/1
  Electronic Gas Pedal RR/1(Motor_Gas_RR) -> E-Motor Mapping RR/2
  Transfer Fcn1/1 -> Gain1/1
  E-Motor Mapping RR/1 -> Transfer Fcn1/1
  Gain1/1 -> Trq_RR/1

== system TV_2018_HIL/CarMaker/IPG Vehicle3/PowerTrain/Electric Powertrain/Gas Pedal ==
  Clock : Clock
  Constant : Constant  Value=0
  Constant1 : Constant
  Fcn : Fcn  Expr=u==0
  Read CM Dict : CarMaker4SL/Read CM Dict  xname=Vhcl.Ignition  xsync=off
  Read CM Dict2 : CarMaker4SL/Read CM Dict  xname=VC.Gas  xsync=off
  Switch : Switch
  Switch1 : Switch
  Write CM Dict : CarMaker4SL/Write CM Dict  xname=Vhcl.Ignition  xsync=off
  VC.Gas : Outport
  wires:
  Read CM Dict2/1 -> Switch/1
  Switch/1 -> VC.Gas/1
  Constant/1 -> Switch/3
  Switch1/1 -> Switch/2, Write CM Dict/1
  Read CM Dict/1 -> Switch1/3
  Constant1/1 -> Switch1/1
  Fcn/1 -> Switch1/2
  Clock/1 -> Fcn/1

== system TV_2018_HIL/CarMaker/Subsystem/Control_System /Power Limit Torque Reduction Controller 2018/Motorestimates ==
  states : Inport
  Ti_lim : Inport  Port=2
  Scope : Scope  NumInputPorts=4
  Scope1 : Scope  NumInputPorts=4
  extractPower2 : MATLAB Function  TreatAsAtomicUnit=on
  motor efficiency table based on RPM and torque{,1..3} (4 alike) : Lookup_n-D  BreakpointsForDimension1=single([1.3,2.7,5.4,7.9,10.4,12.5,14.4,16.0,17.4,18.5,19.6]);  BreakpointsForDimension2=single([500,1000,2000,3000,4000,6000,10000,12000,15000,19000]);  Table=single(reshape([0.6437000036239624,0.5799999833106995,0.44999998807907104,0.3499999940395355,0.28999999165534973,0.23999999463558197,0.20000000298023224,0.17000000178813934,0.14000000059604645,0.12999999523162842,0.10999999940395355,0.7099999785423279,0.699999988079071,0.6100000143051148,0.5099999904632568,0.4399999976158142,0.3799999952316284,0.33000001311302185,0.28999999165534973,0.25,0.2199999988079071,0.20000000298023224,0.7300000190734863,0.7699999809265137,0.7300000190734863,0.6700000166893005,0.6100000143051148,0.550000011920929,0.5,0.44999998807907104,0.4000000059604645,0.36000001430511475,0.33000001311302185,0.7400000095367432,0.800000011920929,0.7900000214576721,0.7400000095367432,0.6899999976158142,0.6399999856948853,0.5899999737739563,0.5400000214576721,0.5,0.46000000834465027,0.41999998688697815,0.75,0.8199999928474426,0.8199999928474426,0.7799999713897705,0.7400000095367432,0.699999988079071,0.6600000262260437,0.6100000143051148,0.5699999928474426,0.5299999713897705,0.49000000953674316,0.7599999904632568,0.8399999737739563,0.8500000238418579,0.8299999833106995,0.800000011920929,0.7699999809265137,0.7400000095367432,0.699999988079071,0.6600000262260437,0.6200000047683716,0.5899999737739563,0.7699999809265137,0.8500000238418579,0.8799999952316284,0.8700000047683716,0.8600000143051148,0.8399999737739563,0.8100000023841858,0.7799999713897705,0.7599999904632568,0.7200000286102295,0.699999988079071,0.7699999809265137,0.8500000238418579,0.8899999856948853,0.8799999952316284,0.8700000047683716,0.8500000238418579,0.8299999833106995,0.8100000023841858,0.7799999713897705,0.7599999904632568,0.7300000190734863,0.7699999809265137,0.8600000143051148,0.8999999761581421,0.8999999761581421,0.8899999856948853,0.8700000047683716,0.8500000238418579,0.8299999833106995,0.8100000023841858,0.7900000214576721,0.6700000166893005,0.7799999713897705,0.8600000143051148,0.8999999761581421,0.9100000262260437,0.8999999761581421,0.8899999856948853,0.8700000047683716,0.8600000143051148,0.8299999833106995,0.7699999809265137,0.699999988079071],11,10));  ExtrapMethod=Clip  UseLastTableValue=on  InternalRulePriority=Speed  RndMeth=Simplest  InputSameDT=on
  Eff_FL : Outport
  Eff_FR : Outport  Port=2
  Eff_RL : Outport  Port=3
  Eff_RR : Outport  Port=4
  wires:
  extractPower2/4(RPM_FR) -> motor efficiency table based on RPM and torque1/2
  motor efficiency table based on RPM and torque/1 -> Scope1/1, Eff_FL/1
  motor efficiency table based on RPM and torque2/1 -> Eff_RL/1
  motor efficiency table based on RPM and torque3/1 -> Eff_RR/1
  Ti_lim/1 -> extractPower2/2(Ti_lim)
  states/1 -> extractPower2/1(states)
  motor efficiency table based on RPM and torque1/1 -> Eff_FR/1
  extractPower2/2(RPM_FL) -> motor efficiency table based on RPM and torque/2
  extractPower2/6(RPM_RL) -> motor efficiency table based on RPM and torque2/2
  extractPower2/1(T_FL) -> Scope/1, motor efficiency table based on RPM and torque/1
  extractPower2/8(RPM_RR) -> motor efficiency table based on RPM and torque3/2
  extractPower2/5(T_RL) -> motor efficiency table based on RPM and torque2/1
  extractPower2/3(T_FR) -> motor efficiency table based on RPM and torque1/1
  extractPower2/7(T_RR) -> motor efficiency table based on RPM and torque3/1

== system TV_2018_HIL/CarMaker/Subsystem/Control_System /Power Limit Torque Reduction Controller 2018/Old powerlimiting  ==
  ti_lim : Inport
  states : Inport  Port=2
  Abs : Abs
  Add : Sum
  Bus Creator : BusCreator  Inputs=4  OutDataTypeStr=Bus: Ti_lim  NonVirtualBus=on
      settings: InheritFromInputs=off
  Bus Selector : BusSelector  OutputSignals=FL,FR,RL,RR
  Discrete PI controller : simulink/Continuous/PID Controller  Controller=PI  TimeDomain=Discrete-time  SampleTime=-1  IntegratorMethod=Forward Euler  FilterMethod=Forward Euler  Form=Parallel  UseFilter=on  ControllerParametersSource=internal  P=powerLimitControl.Kp  I=powerLimitControl.Ki  D=0  N=100  InitialConditionSource=internal  InitialConditionForIntegrator=0  InitialConditionForFilter=0  ExternalReset=none  LimitOutput=on  UpperSaturationLimit=powerLimitControl.upper_sat_limit  LowerSaturationLimit=powerLimitControl.lower_sat_limit  LinearizeAsGain=off  AntiWindupMode=clamping  Kb=settings.Kb_EL;  TrackingMode=off  Kt=1  PParamMin=[]  PParamMax=[]  IParamMin=[]  IParamMax=[]  DParamMin=[]  DParamMax=[]  NParamMin=[]  NParamMax=[]  KbParamMin=[]  KbParamMax=[]  KtParamMin=[]  KtParamMax=[]  POutMin=[]  POutMax=[]  IOutMin=[]  IOutMax=[]  DOutMin=[]  DOutMax=[]  NOutMin=[]  NOutMax=[]  KbOutMin=[]  KbOutMax=[]  KtOutMin=[]  KtOutMax=[]  IntegratorOutMin=[]  IntegratorOutMax=[]  FilterOutMin=[]  FilterOutMax=[]  SumOutMin=[]  SumOutMax=[]  SumI1OutMin=[]  SumI1OutMax=[]  SumI2OutMin=[]  SumI2OutMax=[]  SumI3OutMin=[]  SumI3OutMax=[]  SumDOutMin=[]  SumDOutMax=[]  SaturationOutMin=[]  SaturationOutMax=[]  IntegratorContinuousStateAttributes=''  IntegratorStateMustResolveToSignalObject=off  IntegratorRTWStateStorageClass=Auto  FilterContinuousStateAttributes=''  FilterStateMustResolveToSignalObject=off  FilterRTWStateStorageClass=Auto  DifferentiatorICPrevScaledInput=0  DifferentiatorOutMin=[]  DifferentiatorOutMax=[]
  Negative Power limit : Constant  Value=powerLimitControl.negative_power_limit
  "Positive Power limit " : Constant  Value=powerLimitControl.positive_power_limit
  Product{1..3,5} (4 alike) : Product
  Saturation : Saturate  UpperLimit=1  LowerLimit=0
  Scope : Scope
  Sum : Sum  Inputs=|+-
  Switch : Switch  Criteria=u2 > Threshold
  Switch1 : Switch  Threshold=1
  constant : Constant  Value=single(1)
  constant1 : Constant  Value=powerLimitControl.enable
  constant2 : Constant  Value=single(1)
  exact power : Scope
  extractPower1 : MATLAB Function  TreatAsAtomicUnit=on
  post red fac : Scope
  pre fact : Scope
  "ti_lim " : Outport
  wires:
  Bus Selector/4 -> Product3/2, pre fact/1  "<RR>"
  Bus Selector/1 -> Product5/2  "<FL>"
  Switch1/1 -> Saturation/1
  Bus Selector/2 -> Product2/2  "<FR>"
  Product1/1 -> Bus Creator/3  "RL"
  Discrete PI controller/1 -> Add/2
  Switch/1 -> Sum/1
  Bus Selector/3 -> Product1/2  "<RL>"
  ti_lim/1 -> Bus Selector/1
  Bus Creator/1 -> "ti_lim "/1
  Negative Power limit/1 -> Switch/3
  constant/1 -> Add/1
  Saturation/1 -> Product2/1, Product5/1, Product1/1, Product3/1
  Abs/1 -> Sum/2
  Product2/1 -> Bus Creator/2  "FR"
  "Positive Power limit "/1 -> Switch/1
  Product3/1 -> post red fac/1, Bus Creator/4  "RR"
  extractPower1/1(power) -> Switch/2, exact power/1, Abs/1
  Sum/1 -> Discrete PI controller/1
  states/1 -> extractPower1/1(states)
  Product5/1 -> Bus Creator/1  "FL"
  constant1/1 -> Scope/1, Switch1/2
  constant2/1 -> Switch1/3
  Add/1 -> Switch1/1

== system TV_2018_HIL/CarMaker/Subsystem/Control_System /Slip Rate Control /SMC Traction Control ==
  note: Tc ouput is either an increase or decrease in torque .
  states : Inport
  Ti_ref : Inport  Port=2
  T_requested : Inport  Port=3
  Bus Selector : BusSelector  OutputSignals=FL,FR,RL,RR
  Constant : Constant  Value=tractionControl.Kp
  Constant1 : Constant  Value=tractionControl.Ki
  Constant2 : Constant  Value=tractionControl.Slip_ratio_ref
  Gain : Gain  Gain=single(3.6)
  Gain2 : Gain  Gain=single(3.6)
  Ki Loopup : Lookup_n-D  NumberOfTableDimensions=1  BreakpointsForDimension1=[0 5 10]  Table="[tractionControl.Ki_start tractionControl.Ki_middle  tractionControl.Ki_end]*tractionControl.Ki_scaling"  ExtrapMethod=Clip  UseLastTableValue=on  InternalRulePriority=Speed  RndMeth=Simplest  InputSameDT=on
  Kp Lookup : Lookup_n-D  NumberOfTableDimensions=1  BreakpointsForDimension1="[0  5]"  Table="[tractionControl.Kp_start  tractionControl.Kp_end]*tractionControl.Kp_scaling"  ExtrapMethod=Clip  UseLastTableValue=on  InternalRulePriority=Speed  RndMeth=Simplest  InputSameDT=on
  MATLAB Function : MATLAB Function  TreatAsAtomicUnit=on
  MATLAB Function1 : MATLAB Function  TreatAsAtomicUnit=on
  Slip Rate FL : Subsystem
  Slip Rate FL1 : Subsystem
  Slip Rate FL2 : Subsystem
  Slip Rate FL3 : Subsystem
  Ti_SR : Outport
  wires:
  states/1 -> MATLAB Function1/1(states), Slip Rate FL/4(states), Slip Rate FL1/4(states), Slip Rate FL2/4(states), Slip Rate FL3/4(states), MATLAB Function/9(states)
  Ti_ref/1 -> Bus Selector/1
  Bus Selector/1 -> [Ti_FL]  "<FL>"
  Bus Selector/2 -> [Ti_FR]  "<FR>"
  Bus Selector/3 -> [Ti_RL]  "<RL>"
  Bus Selector/4 -> [Ti_RR]  "<RR>"
  [SR_Kp] -> Slip Rate FL/2(Kp)
  Kp Lookup/1 -> ?
  Ki Loopup/1 -> [SR_Ki]
  Gain/1 -> Kp Lookup/1
  Gain2/1 -> Ki Loopup/1
  Constant1/1 -> ?
  Constant/1 -> [SR_Kp]
  MATLAB Function/1(Ti_lim) -> Ti_SR/1
  [Ti_FL] -> MATLAB Function/1(Ti_FL)
  [Ti_RR] -> MATLAB Function/4(Ti_RR)
  [Ti_RL] -> MATLAB Function/3(Ti_RL)
  [Ti_FR] -> MATLAB Function/2(Ti_FR)
  T_requested/1 -> MATLAB Function/10(T_req)
  MATLAB Function1/1(SR_FL) -> Slip Rate FL/3(SR)
  Constant2/1 -> Slip Rate FL3/1(SR_ref), Slip Rate FL2/1(SR_ref), Slip Rate FL1/1(SR_ref), Slip Rate FL/1(SR_ref)
  MATLAB Function1/5(vx) -> Gain2/1, Gain/1
  MATLAB Function1/2(SR_FR) -> Slip Rate FL1/3(SR)
  MATLAB Function1/3(SR_RL) -> Slip Rate FL2/3(SR)
  MATLAB Function1/4(SR_RR) -> Slip Rate FL3/3(SR)
  [SR_Kp] -> Slip Rate FL1/2(Kp)
  [SR_Kp] -> Slip Rate FL2/2(Kp)
  [SR_Kp] -> Slip Rate FL3/2(Kp)
  Slip Rate FL/1(Tc) -> MATLAB Function/5(TC_FL)
  Slip Rate FL1/1(Tc) -> MATLAB Function/6(TC_FR)
  Slip Rate FL2/1(Tc) -> MATLAB Function/7(TC_RL)
  Slip Rate FL3/1(Tc) -> MATLAB Function/8(TC_RR)

== system TV_2018_HIL/CarMaker/Subsystem/Control_System /Slip Rate Control /SUM ==
  note: consider to scale FL&FR for steer angle
  In1 : Inport
  Bus Selector : BusSelector  OutputSignals=FL,FR,RL,RR
  Sum : Sum  Inputs=|++
  Sum1 : Sum  Inputs=|++
  Sum2 : Sum  Inputs=|++
  Out1 : Outport
  wires:
  In1/1 -> Bus Selector/1
  Bus Selector/1 -> Sum/1  "<FL>"
  Bus Selector/2 -> Sum1/1  "<FR>"
  Bus Selector/3 -> Sum2/1  "<RL>"
  Bus Selector/4 -> Sum2/2  "<RR>"
  Sum2/1 -> Sum1/2
  Sum1/1 -> Sum/2
  Sum/1 -> Out1/1

== system TV_2018_HIL/CarMaker/Subsystem/Control_System /Slip Rate Control /Traction Controllers ==
  states : Inport
  Ti_ref : Inport  Port=2
  T_requested : Inport  Port=3
  Bus Selector : BusSelector  OutputSignals=FL,FR,RL,RR
  Constant2 : Constant  Value=tractionControl.Slip_ratio_ref
  MATLAB Function : MATLAB Function  TreatAsAtomicUnit=on
  MATLAB Function1 : MATLAB Function  TreatAsAtomicUnit=on
  Mux18 : Mux
  Slip Rate FL : Subsystem
  Slip Rate FR : Subsystem
  Slip Rate RL : Subsystem
  Slip Rate RR : Subsystem
  tcOutput : Scope
  tcOutput1 : Scope  NumInputPorts=4
  Ti_SR : Outport
  wires:
  states/1 -> MATLAB Function1/1(states), MATLAB Function/9(states)
  Ti_ref/1 -> MATLAB Function1/3(T_tv), Bus Selector/1
  Bus Selector/1 -> [Ti_FL]  "<FL>"
  Bus Selector/2 -> [Ti_FR]  "<FR>"
  Bus Selector/3 -> [Ti_RL]  "<RL>"
  Bus Selector/4 -> [Ti_RR]  "<RR>"
  [Ti_FL] -> Slip Rate FL/5(Ti_ref)
  [Ti_FR] -> Slip Rate FR/5(Ti_ref)
  [Ti_RL] -> Slip Rate RL/5(Ti_ref)
  [Ti_RR] -> Slip Rate RR/5(Ti_ref)
  [SR_Ki] -> Slip Rate FL/3(Ki)
  [SR_Kp] -> Slip Rate FL/2(Kp)
  [SR_Kp] -> Slip Rate FR/2(Kp)
  [SR_Ki] -> Slip Rate FR/3(Ki)
  [SR_Kp] -> Slip Rate RL/2(Kp)
  [SR_Ki] -> Slip Rate RL/3(Ki)
  [SR_Kp] -> Slip Rate RR/2(Kp)
  [SR_Ki] -> Slip Rate RR/3(Ki)
  Slip Rate FL/1(TC_output) -> Mux18/1, MATLAB Function/5(TC_FL)  "FL"
  Slip Rate FR/1(TC_output) -> Mux18/2, MATLAB Function/6(TC_FR)  "FR"
  Slip Rate RR/1(TC_output) -> Mux18/4, MATLAB Function/8(TC_RR)  "RR"
  Slip Rate RL/1(TC_output) -> Mux18/3, MATLAB Function/7(TC_RL)  "RL"
  MATLAB Function/1(Ti_lim) -> Ti_SR/1
  [Ti_FL] -> MATLAB Function/1(Ti_FL)
  [Ti_RR] -> MATLAB Function/4(Ti_RR)
  [Ti_RL] -> MATLAB Function/3(Ti_RL)
  [Ti_FR] -> MATLAB Function/2(Ti_FR)
  T_requested/1 -> MATLAB Function1/2(T_req), MATLAB Function/10(T_req)
  MATLAB Function1/2(SR_FR) -> tcOutput1/2, Slip Rate FR/4(SR)
  MATLAB Function1/3(SR_RL) -> tcOutput1/3, Slip Rate RL/4(SR)
  Constant2/1 -> Slip Rate RL/1(SR_ref), Slip Rate FR/1(SR_ref), Slip Rate FL/1(SR_ref), Slip Rate RR/1(SR_ref)
  MATLAB Function1/1(SR_FL) -> tcOutput1/1, Slip Rate FL/4(SR)
  MATLAB Function1/5(Kp) -> [SR_Kp]
  MATLAB Function1/6(Ki) -> [SR_Ki]
  Mux18/1 -> tcOutput/1
  MATLAB Function1/4(SR_RR) -> tcOutput1/4, Slip Rate RR/4(SR)
